simulink model "NIRM3"  (R2022b)
settings: Solver=VariableStepAuto  StartTime=0.0  StopTime=90  RelTol=1e-3
settings Model: Creator=nazarcooltaev  LastModifiedBy=nazarcooltaev

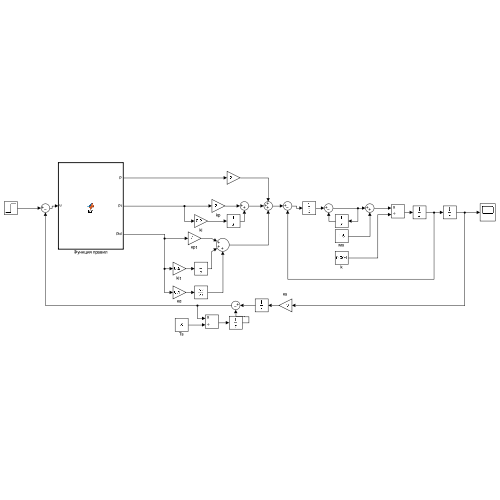
[thumbnail: Simulink's stored preview of the top-level diagram]
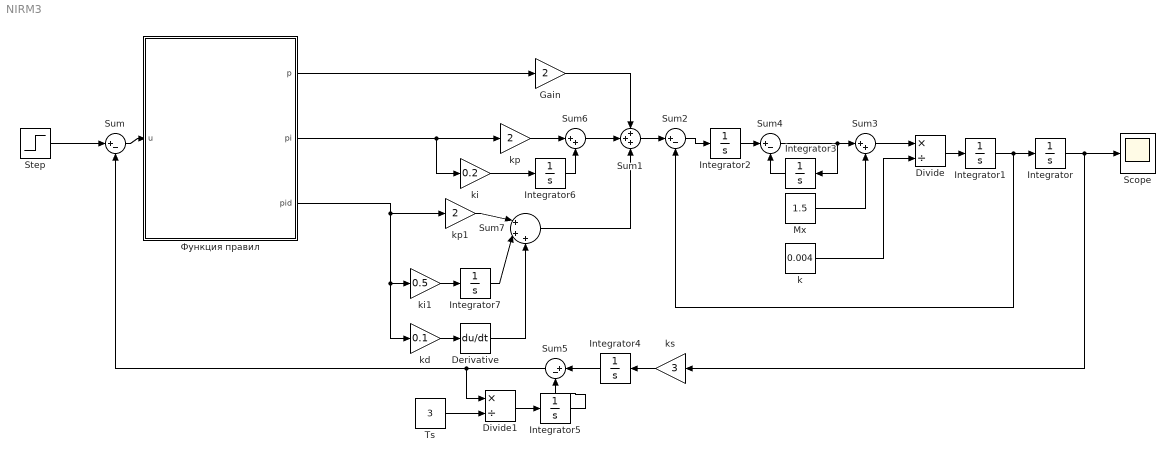
== system NIRM3 ==
  Derivative : Derivative
  Divide : Product  Inputs=*/
  Divide1 : Product  Inputs=*/
  Gain : Gain  Gain=2
  Integrator{,1..7} (8 alike) : Integrator
  Mx : Constant  Value=1.5
  Scope : Scope
  Step : Step  Time=2  SampleTime=0
  Sum{,2,4..5} (4 alike) : Sum  Inputs=|+-
  Sum1 : Sum  Inputs=+++
  Sum3 : Sum  Inputs=|++
  Sum6 : Sum  Inputs=|++
  Sum7 : Sum  Inputs=|+++
  Ts : Constant  Value=3
  k : Constant  Value=0.004
  kd : Gain  Gain=0.1
  ki : Gain  Gain=0.2
  ki1 : Gain  Gain=0.5
  kp : Gain  Gain=2
  kp1 : Gain  Gain=2
  ks : Gain  Gain=3
  Функция правил : MATLAB Function  TreatAsAtomicUnit=on
  wires:
  Step/1 -> Sum/1
  Sum/1 -> Функция правил/1(u)
  Функция правил/1(p) -> Gain/1
  Sum5/1 -> Divide1/1, Sum/2
  Integrator/1 -> ks/1, Scope/1
  Sum2/1 -> Integrator2/1
  Integrator1/1 -> Integrator/1, Sum2/2
  Sum7/1 -> Sum1/3
  Gain/1 -> Sum1/1
  Sum6/1 -> Sum1/2
  Sum1/1 -> Sum2/1
  Divide/1 -> Integrator1/1
  Sum3/1 -> Divide/1
  Mx/1 -> Sum3/2
  k/1 -> Divide/2
  Integrator2/1 -> Sum4/1
  Integrator3/1 -> Sum4/2
  Sum4/1 -> Integrator3/1, Sum3/1
  ks/1 -> Integrator4/1
  Ts/1 -> Divide1/2
  Integrator4/1 -> Sum5/1
  Divide1/1 -> Integrator5/1
  Integrator5/1 -> Sum5/2
  Функция правил/2(pi) -> ki/1, kp/1
  kp/1 -> Sum6/1
  Integrator6/1 -> Sum6/2
  ki/1 -> Integrator6/1
  kp1/1 -> Sum7/1
  ki1/1 -> Integrator7/1
  Функция правил/3(pid) -> kd/1, ki1/1, kp1/1
  Integrator7/1 -> Sum7/2
  Derivative/1 -> Sum7/3
  kd/1 -> Derivative/1

== matlab function NIRM3/Функция правил ==
  data: u input; p output; pi output; pid output
function [p, pi, pid] = fcn(u)

p = 0;
  pi = 0;
  pid = 0;
if abs(u) < 0.5
  p = 0;
  pi = 0;
  pid = u;
elseif abs(u) >= 0.5 && abs(u) < 0.7
  p = 0;
  pi = u;
  pid = 0;
elseif abs(u) >= 0.7
  p = u;
  pi = 0;
  pid = 0;
end
